simulink model "lorenz_sim"  (Simulink 10.2)
settings: Solver=ode4  StartTime=0.0  StopTime=5  FixedStep=0.01  RelTol=1e-3  EnableMultiTasking=on
values from neighbouring files (symbols this model uses):
  b = 8/3    (= 2.66666666667)    [main.m]
  delt = 10    [main.m]
  r = 20    [main.m]
  x0 = 1    [main.m]
  y0 = 1    [main.m]
  z0 = 1    [main.m]
settings Model: Creator=jiangdonghua  ModifiedByFormat=zhl_chosenone  LastModifiedBy=zhl_chosenone
settings DataIOCC: LimitDataPoints=on
settings OptimizationCC: InitFltsAndDblsToZero=on
settings DebuggingCC: SaveWithParameterizedLinksMsg=none  SignalResolutionControl=TryResolveAllWithWarning  SolverPrmCheckMsg=warning  MultiTaskDSMMsg=warning  MultiTaskCondExecSysMsg=none
settings SFSimCC: SimUseLocalCustomCode=on  CustomCodeUndefinedFunction=FilterOut
settings RTWCC: RTWUseLocalCustomCode=on
settings GRTTargetCC: TargetFcnLib=ansi_tfl_tmw.mat
settings ConfigComp: CovExternalEMLEnable=on

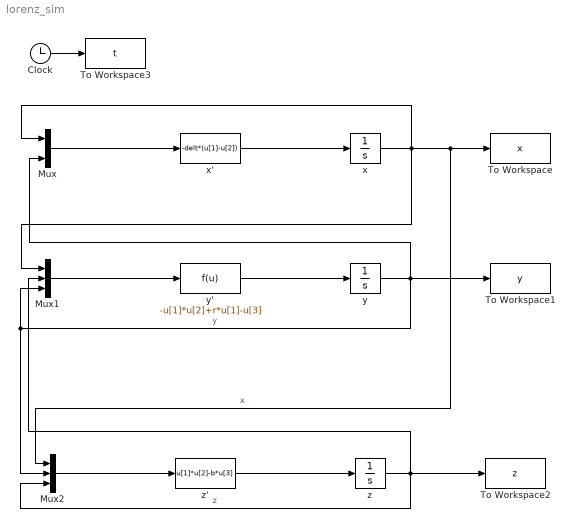
== system lorenz_sim ==
  Clock : Clock
  Mux : Mux  Inputs=2
  Mux1 : Mux  Inputs=3
  Mux2 : Mux  Inputs=3
  To Workspace : ToWorkspace  VariableName=x  SampleTime=-1
  To Workspace1 : ToWorkspace  VariableName=y  SampleTime=-1
  To Workspace2 : ToWorkspace  VariableName=z  SampleTime=-1
  To Workspace3 : ToWorkspace  VariableName=t  SampleTime=-1
  x : Integrator  InitialCondition=x0
  x' : Fcn  Expr=-delt*(u[1]-u[2])
  y : Integrator  InitialCondition=y0
  y' : Fcn  Expr=-u[1]*u[2]+r*u[1]-u[3]
  z : Integrator  InitialCondition=z0
  z' : Fcn  Expr=u[1]*u[2]-b*u[3]
  wires:
  Mux/1 -> x'/1
  x'/1 -> x/1
  Mux1/1 -> y'/1
  y'/1 -> y/1
  Mux2/1 -> z'/1
  z'/1 -> z/1
  x/1 -> Mux/1, To Workspace/1, Mux2/1, Mux1/1  "x"
  y/1 -> Mux1/3, Mux2/2, To Workspace1/1, Mux/2  "y"
  z/1 -> Mux2/3, To Workspace2/1, Mux1/2  "z"
  Clock/1 -> To Workspace3/1
